simulink model "kaerman"  (R2016a)
settings: Solver=ode45  StartTime=0.0  StopTime=10  RelTol=1e-3
undefined symbols (not defined in the file or in its folder): kaerman1
libraries: simulink x1
settings Model: ExtModeTrigMode=oneshot  ExtModeArmWhenConnect=off  Creator=hp  LastModifiedBy=Administrator
settings DataIOCC: SaveFormat=Array  SignalLoggingSaveFormat=ModelDataLogs
settings OptimizationCC: BlockReduction=off  BooleanDataType=off  InitFltsAndDblsToZero=on
settings DebuggingCC: SaveWithParameterizedLinksMsg=none  UnderspecifiedInitializationDetection=Classic  MergeDetectMultiDrivingBlocksExec=none  SignalResolutionControl=TryResolveAllWithWarning  MultiTaskDSMMsg=warning  MultiTaskCondExecSysMsg=none  FcnCallInpInsideContextMsg=UseLocalSettings
settings HardwareCC: ProdBitPerPointer=32  ProdLargestAtomicFloat=None  ProdIntDivRoundTo=Undefined  ProdEndianess=Unspecified  ProdWordSize=32  ProdHWDeviceType=32-bit Generic  TargetUnknown=on
settings ModelReferenceCC: PropagateSignalLabelsOutOfModel=off
settings GRTTargetCC: TargetFcnLib=ansi_tfl_tmw.mat  GeneratePreprocessorConditionals=Use local settings  CombineOutputUpdateFcns=off  GRTInterface=on
settings ConfigComp: CovModelRefEnable=Off

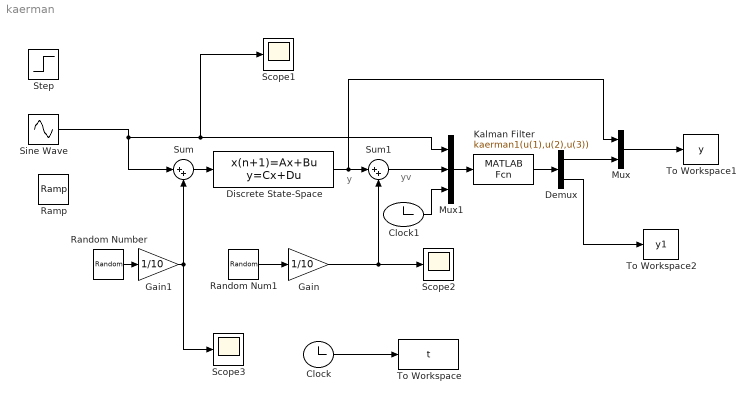
== system kaerman ==
  note: y
  note: yv
  Clock : Clock
  Clock1 : Clock
  Demux : Demux  Outputs=2
  Discrete State-Space : DiscreteStateSpace  A=[1.0000 0.0010;0 0.9753]  B=[0.0001;0.1314]  C=[1 0]  D=0  SampleTime=0.001
  Gain : Gain  Gain=1/10  SaturateOnIntegerOverflow=on  OutDataTypeStr=Inherit: Same as input  ParamDataTypeStr=Inherit: Same as input
  Gain1 : Gain  Gain=1/10  SaturateOnIntegerOverflow=on  OutDataTypeStr=Inherit: Same as input  ParamDataTypeStr=Inherit: Same as input
  Kalman Filter : MATLABFcn  MATLABFcn=kaerman1(u(1),u(2),u(3))  OutputDimensions=2
  Mux : Mux  Inputs=2
  Mux1 : Mux  Inputs=3
  Ramp : simulink/Sources/Ramp  slope=0.005  start=0  X0=0
  Random Num1 : RandomNumber  SampleTime=0.001
  Random Number : RandomNumber  SampleTime=0.001
  Scope1 : Scope
  Scope2 : Scope
  Scope3 : Scope
  Sine Wave : Sin  SampleTime=0
  Step : Step  SampleTime=1
  Sum : Sum  Inputs=|++  SaturateOnIntegerOverflow=on  InputSameDT=on  OutDataTypeStr=Inherit: Same as first input
  Sum1 : Sum  Inputs=|++  SaturateOnIntegerOverflow=on  InputSameDT=on  OutDataTypeStr=Inherit: Same as first input
  To Workspace : ToWorkspace  VariableName=t  SampleTime=-1
  To Workspace1 : ToWorkspace  VariableName=y  SampleTime=-1
  To Workspace2 : ToWorkspace  VariableName=y1  SampleTime=-1
  wires:
  Mux1/1 -> Kalman Filter/1
  Clock1/1 -> Mux1/3
  Sum/1 -> Discrete State-Space/1
  Sum1/1 -> Mux1/2
  Discrete State-Space/1 -> Mux/1, Sum1/1
  Random Number/1 -> Gain1/1
  Kalman Filter/1 -> Demux/1
  Gain1/1 -> Sum/2, Scope3/1
  Random Num1/1 -> Gain/1
  Gain/1 -> Sum1/2, Scope2/1
  Demux/2 -> To Workspace2/1
  Demux/1 -> Mux/2
  Clock/1 -> To Workspace/1
  Mux/1 -> To Workspace1/1
  Sine Wave/1 -> Scope1/1, Mux1/1, Sum/1
